simulink model "nova_validacao"  (R2018a)
settings: Solver=FixedStepAuto  StartTime=0.0  StopTime=22  FixedStep=0.01  RelTol=1e-3
undefined symbols (not defined in the file): tf5, tf6, tf7
libraries: arduino_io_lib x5
settings Model: Creator=Mauricio  LastModifiedBy=Mauricio

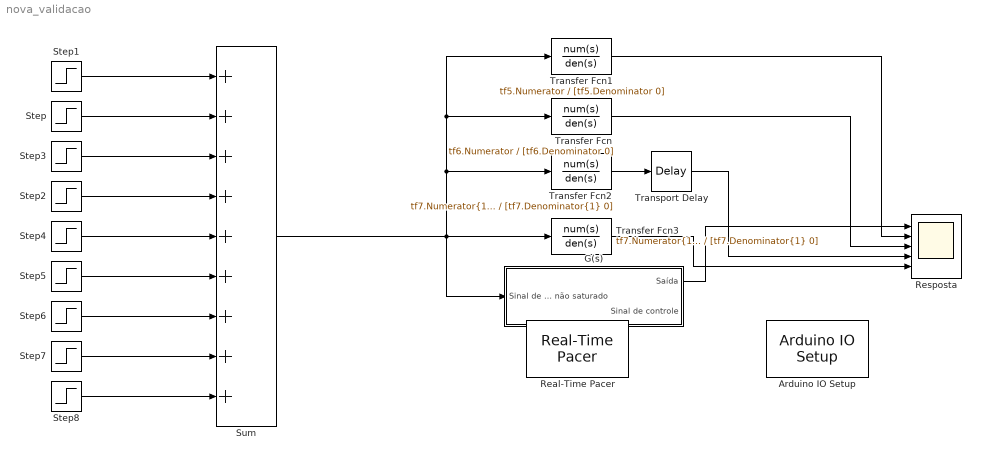
== system nova_validacao ==
  Arduino IO Setup : arduino_io_lib/Arduino IO Setup  Priority=3  arduinoVar=Temporary arduino variable: Arduino1  workspaceVarName=a  comPort=COM4
  "G(s) " : Subsystem
  Real-Time Pacer : arduino_io_lib/Real-Time Pacer  simTimePerRealTime=1
  Resposta : Scope  NumInputPorts=5
  Step : Step  Time=7.9  After=-100  SampleTime=0.05
  Step1 : Step  Time=5  After=50  SampleTime=0.05
  Step2 : Step  Time=11+1.5  After=100  SampleTime=0.05
  Step3 : Step  Time=11  After=50  SampleTime=0.05
  Step4 : Step  Time=11+2.9  After=-200  SampleTime=0.05
  Step5 : Step  Time=11+4.5  After=100  SampleTime=0.05
  Step6 : Step  Time=15.5+2  After=75  SampleTime=0.05
  Step7 : Step  Time=15.5+3.9  After=-150  SampleTime=0.05
  Step8 : Step  Time=15.5+6  After=75  SampleTime=0.05
  Sum : Sum  Inputs=+++++++++
  Transfer Fcn : TransferFcn  Numerator=tf6.Numerator  Denominator=[tf6.Denominator 0]
  Transfer Fcn1 : TransferFcn  Numerator=tf5.Numerator  Denominator=[tf5.Denominator 0]
  Transfer Fcn2 : TransferFcn  Numerator=tf7.Numerator{1}  Denominator=[tf7.Denominator{1} 0]
  Transfer Fcn3 : TransferFcn  Numerator=tf7.Numerator{1}  Denominator=[tf7.Denominator{1} 0]
  Transport Delay : TransportDelay  DelayTime=0.03648
  wires:
  Step1/1 -> Sum/1
  Step/1 -> Sum/2
  Step3/1 -> Sum/3
  Step2/1 -> Sum/4
  Step4/1 -> Sum/5
  Step5/1 -> Sum/6
  Step6/1 -> Sum/7
  Step7/1 -> Sum/8
  Step8/1 -> Sum/9
  Transfer Fcn/1 -> Resposta/3
  Transfer Fcn1/1 -> Resposta/2
  Transfer Fcn2/1 -> Transport Delay/1
  Transport Delay/1 -> Resposta/4
  Sum/1 -> Transfer Fcn3/1, Transfer Fcn2/1, Transfer Fcn1/1, Transfer Fcn/1, "G(s) "/1(Sinal de controle não saturado)
  Transfer Fcn3/1 -> Resposta/5
  "G(s) "/1(Saída) -> Resposta/1

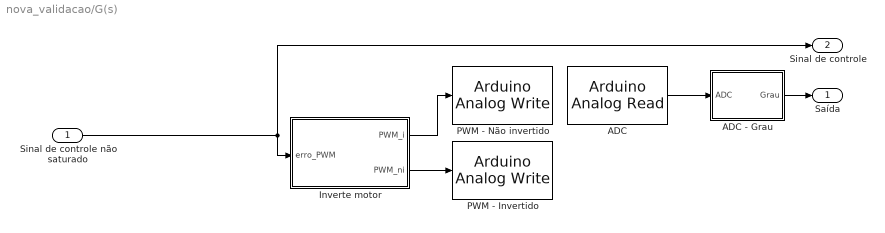
== system nova_validacao/G(s)  ==
  Sinal de controle não saturado : Inport
  ADC : arduino_io_lib/Arduino Analog Read  arduinoVar=Temporary arduino variable: Arduino1  arduinoPin=2  T=0.01
  ADC - Grau : MATLAB Function  TreatAsAtomicUnit=on
  Inverte motor : MATLAB Function  TreatAsAtomicUnit=on
  PWM - Invertido : arduino_io_lib/Arduino Analog Write  arduinoVar=Temporary arduino variable: Arduino1  arduinoPin=6  T=0.05
  PWM - Não invertido : arduino_io_lib/Arduino Analog Write  arduinoVar=Temporary arduino variable: Arduino1  arduinoPin=5  T=0.05
  Saída : Outport
  Sinal de controle : Outport  Port=2
  wires:
  ADC/1 -> ADC - Grau/1(ADC)
  Inverte motor/2(PWM_ni) -> PWM - Invertido/1
  Inverte motor/1(PWM_i) -> PWM - Não invertido/1
  ADC - Grau/1(Grau) -> Saída/1
  Sinal de controle não saturado/1 -> Sinal de controle/1, Inverte motor/1(erro_PWM)

== matlab function nova_validacao/G(s) /ADC - Grau ==
  data: ADC input; Grau output
function Grau = fcn(ADC)
Grau = -0.17413322126497163269594452616096*ADC + 136.2690584156335364572389157386;

== matlab function nova_validacao/G(s) /Inverte motor ==
  data: PWM_i output; PWM_ni output; erro_PWM input
function [PWM_i, PWM_ni] = fcn(erro_PWM)
dead_zone = 45;
%erro_permissivel = 0.5;

%Confere se a saída está dentro de um erro aceitável, já que não tem
%integrador no controlador
%if(abs(erro) <= erro_permissivel)
 %   erro_PWM = 0;
%end

%DESLIGADO
if(erro_PWM == 0)
    PWM_ni = 0;
    PWM_i = 0;
%REVERSO
elseif(erro_PWM>0)
    erro_PWM = erro_PWM + dead_zone; 
    PWM_i = erro_PWM;
    PWM_ni = 0;
%FRENTE
else
    erro_PWM = erro_PWM - dead_zone;
    PWM_ni = abs(erro_PWM);
    PWM_i = 0;
end
